simulink model "actuation"  (R2022a)
settings: Solver=FixedStepAuto  StartTime=0.0  StopTime=10.0  RelTol=1e-3
libraries: arduinolib x4, simulink x3
settings Model: ExtModeTrigDuration=2  Creator=daixingze  LastModifiedBy=daixingze
settings OptimizationCC: EnhancedBackFolding=on  PassReuseOutputArgsAs=Individual arguments  ZeroExternalMemoryAtStartup=off  ZeroInternalMemoryAtStartup=off  MaxStackSize=64  OptimizeBlockOrder=speed  DifferentSizesBufferReuse=on  OptimizationCustomize=off  EfficientTunableParamExpr=on
settings DebuggingCC: ParameterTunabilityLossMsg=error
settings HardwareCC: ProdBitPerInt=16  ProdBitPerPointer=16  ProdBitPerSizeT=16  ProdBitPerPtrDiffT=16  ProdLargestAtomicFloat=None  ProdWordSize=8  ProdHWDeviceType=Atmel->AVR
settings SFSimCC: MATLABDynamicMemAlloc=off
settings RTWCC: SystemTargetFile=ert.tlc  HardwareBoard=Arduino Mega 2560  TemplateMakefile=ert_default_tmf  Toolchain=Arduino AVR
settings CodeAppCC: ForceParamTrailComments=on  IgnoreCustomStorageClasses=off  OperatorAnnotations=on  SimulinkDataObjDesc=on  SFDataObjDesc=on  InsertBlockDesc=on
settings ERTTargetCC: SupportContinuousTime=on  SupportVariableSizeSignals=on  ExtModeTransport=3  ExtModeStaticAlloc=on  ExtModeStaticAllocSize=2048  ExtModeMexFile=ext_xcp  ExtModeIntrfLevel=Level2 - Open

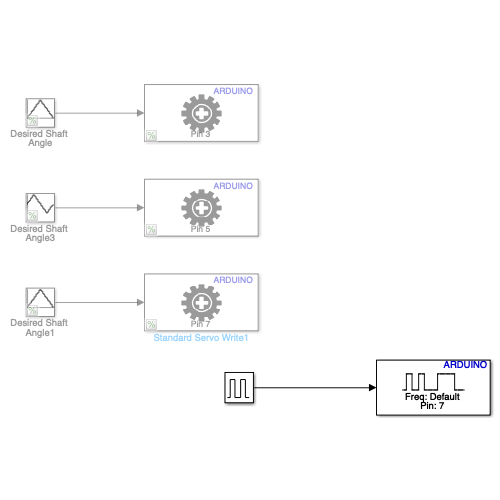
[thumbnail: Simulink's stored preview of the top-level diagram]
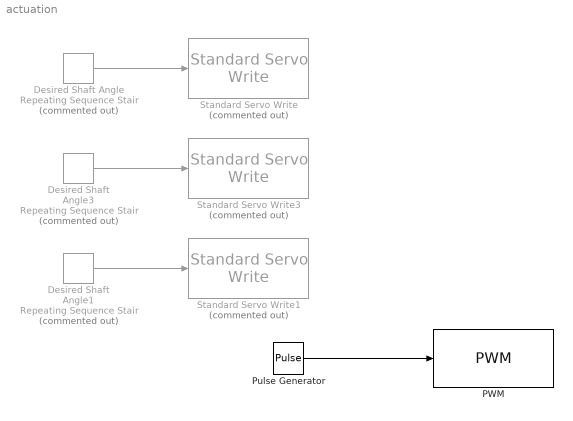
== system actuation ==
  Desired Shaft Angle : simulink/Sources/Repeating Sequence Stair  Commented=on  OutValues=[0:180 179:-1:1]  tsamp=0.01  OutMin=[]  OutMax=[]  OutDataTypeStr=uint8  OutputDataTypeScalingMode=uint8  OutDataType=fixdt(0,8)  ConRadixGroup=Best Precision: Vector-wise  OutScaling=2^-12
  Desired Shaft Angle1 : simulink/Sources/Repeating Sequence Stair  Commented=on  OutValues=[0:90 90:-1:1]  tsamp=0.01  OutMin=[]  OutMax=[]  OutDataTypeStr=uint8  OutputDataTypeScalingMode=uint8  OutDataType=fixdt(0,8)  ConRadixGroup=Best Precision: Vector-wise  OutScaling=2^-12
  Desired Shaft Angle3 : simulink/Sources/Repeating Sequence Stair  Commented=on  OutValues=[45:90 90:-1:1 1:45]  tsamp=0.01  OutMin=[]  OutMax=[]  OutDataTypeStr=uint8  OutputDataTypeScalingMode=uint8  OutDataType=fixdt(0,8)  ConRadixGroup=Best Precision: Vector-wise  OutScaling=2^-12
  PWM : arduinolib/PWM  pinNumber=7  frequencyType=Default  desiredFrequency=490.2  achievableFrequency=490.2
  Pulse Generator : DiscretePulseGenerator  PulseType=Time based  Period=0.001  PulseWidth=50
  Standard Servo Write : arduinolib/Standard Servo Write  Commented=on  pinNumber=3  ServoIndex=0  blockPlatform=arduino
  Standard Servo Write1 : arduinolib/Standard Servo Write  Commented=on  pinNumber=7  ServoIndex=1  blockPlatform=arduino
  Standard Servo Write3 : arduinolib/Standard Servo Write  Commented=on  pinNumber=5  ServoIndex=2  blockPlatform=arduino
  wires:
  Desired Shaft Angle/1 -> Standard Servo Write/1
  Desired Shaft Angle1/1 -> Standard Servo Write1/1
  Pulse Generator/1 -> PWM/1
  Desired Shaft Angle3/1 -> Standard Servo Write3/1
